simulink model "untitled"  (R2022b)
settings: Solver=ode1  StartTime=0.0  StopTime=1e4  FixedStep=0.01  RelTol=1e-3
libraries: simulink x1, simulink_extras x1
settings Model: Creator=asus  LastModifiedBy=asus

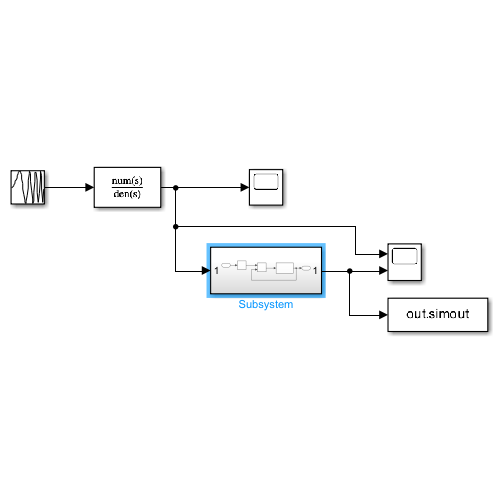
[thumbnail: Simulink's stored preview of the top-level diagram]
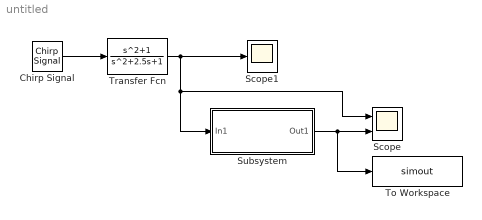
== system untitled ==
  Chirp Signal : simulink/Sources/Chirp Signal  f1=0.01/(2*pi)  T=1e4  f2=100/(2*pi)
  Scope : Scope  NumInputPorts=2
  Scope1 : Scope
  Subsystem : Subsystem
  To Workspace : ToWorkspace  VariableName=simout  SampleTime=-1
  Transfer Fcn : TransferFcn  Numerator=[1 0 1]  Denominator=[1 2.5 1]
  wires:
  Chirp Signal/1 -> Transfer Fcn/1
  Transfer Fcn/1 -> Scope/1, Subsystem/1(In1), Scope1/1
  Subsystem/1(Out1) -> To Workspace/1, Scope/2

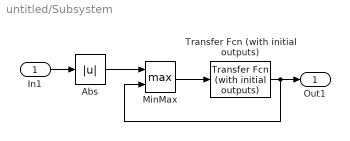
== system untitled/Subsystem ==
  In1 : Inport
  Abs : Abs  SaturateOnIntegerOverflow=off
  MinMax : MinMax  Function=max  Inputs=2
  Transfer Fcn (with initial outputs) : simulink_extras/Additional Linear/Transfer Fcn (with initial outputs)  N=[0.9]  D="[1  1]"  Y0=1  U0=0
  Out1 : Outport
  wires:
  Abs/1 -> MinMax/1
  MinMax/1 -> Transfer Fcn (with initial outputs)/1
  Transfer Fcn (with initial outputs)/1 -> MinMax/2, Out1/1
  In1/1 -> Abs/1
